simulink model "ADCS_onOrbit_14_4_3"  (R2024b)
settings: Solver=ode4  StartTime=0.0  StopTime=tspan  FixedStep=1  RelTol=1e-5
values from neighbouring files (symbols this model uses):
  A_list = [10*30; 10*30; 10*10; 10*30; 10*30; 10*10] * 1e-04    [acsLoadParameters.m]
  A_m = eye(3)    [acsLoadParameters.m]
  A_w = eye(3)    [acsLoadParameters.m]
  CD = 2.3    [acsLoadParameters.m]
  COP = [xAxis/2   0          0 ... (first row only)    [acsLoadParameters.m]
  dYear = decyear(YYYY,MM,DD)    [acsLoadParameters.m]
  e = 6.91944e-15    [acsLoadParameters.m]
  eta = 0.3    [acsLoadParameters.m]
  inc = 97.4065    [acsLoadParameters.m]
  J_body = [I_x 0 0; 0 I_y 0; 0 0 I_z]    [acsLoadParameters.m]
  J_wheels = [12894 0 0; 0 12774 0; 0 0 18389] * 1e-09    [acsLoadParameters.m]
  JD0 = juliandate(YYYY,MM,DD,HH,MIN,SEC)    [acsLoadParameters.m]
  K_d = 0.008    [acsLoadParameters.m]
  K_p = 0.003    [acsLoadParameters.m]
  K_w = 50e4    (= 500000)    [acsLoadParameters.m]
  m = 4    [acsLoadParameters.m]
  mag_moment = [0.005; 0.005; 0.005]    [acsLoadParameters.m]
  mu = 398600.4418    [acsLoadParameters.m]
  n_list = [1 0 0; 0 1 0; 0 0 1; -1 0 0; 0 -1 0; 0 0 -1]    [acsLoadParameters.m]
  omega = 0    [acsLoadParameters.m]    (also in orbit_plot_sfcn.m = block.InputPort(4).Data(:))
  p = 0.00000451    (= 4.51e-06)    [acsLoadParameters.m]    (also in cubesat_attitude_sfcn.m = ud.cubePos)
  P_0 = 0.0000001 * eye(7)    [acsLoadParameters.m]
  period = sqrt((4* pi^2 * semimajor_axis^3)/(mu))    [acsLoadParameters.m]
  q_ini = [0; 0; 0; 1]    [acsLoadParameters.m]
  raan = 132.112    [acsLoadParameters.m]
  rE = 6378.14    [acsLoadParameters.m]
  semimajor_axis = rE + h_apogee    (= 6898.14)    [acsLoadParameters.m]
  sigma_B_b = 0.05 * [1; 1; 1]    [acsLoadParameters.m]
  sigma_drift = 0.05 * [1; 1; 1] * 0    [acsLoadParameters.m]
  sigma_n = (0.05) * [1; 1; 1] * 0    [acsLoadParameters.m]
  sigma_S_b = 0.05 * [1; 1; 1]    [acsLoadParameters.m]
  tau = 300    [ATT_EKF_DOT.m]    (also in acsLoadParameters.m)
  true_anomaly = 1.42146e-14    [acsLoadParameters.m]
  w_b_ini = [0; 0.1; 0.1]    [acsLoadParameters.m]
  w_bias_0 = 0.0001 * [1; 1; 1] * 0    [acsLoadParameters.m]
  w_w_ini = [0; 0; 0]    [acsLoadParameters.m]
  wE = [0 0 15.04*(pi/180)*(1/3600)]    [acsLoadParameters.m]
undefined symbols (not defined in the file or in its folder): WMM2020
libraries: simulink_extras x13, matrix_library x9, sharedtransform x7, aerolibgravity2 x1, aerolibutil x1
(part 1 of 3)
settings Model: SimulationMode=accelerator  Creator=nimis  LastModifiedBy=nimis
settings SolverCC: AlgebraicLoopSolver=TrustRegion
settings DebuggingCC: AlgebraicLoopMsg=none

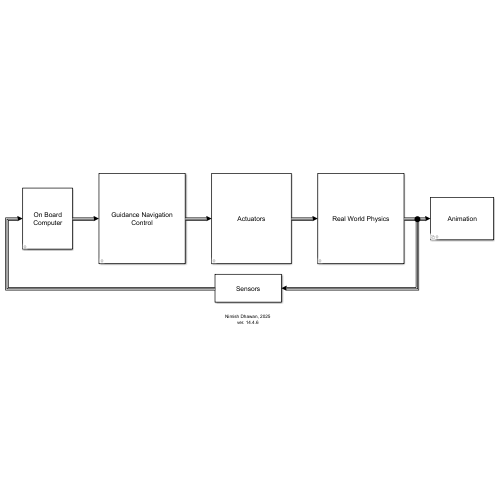
[thumbnail: Simulink's stored preview of the top-level diagram]
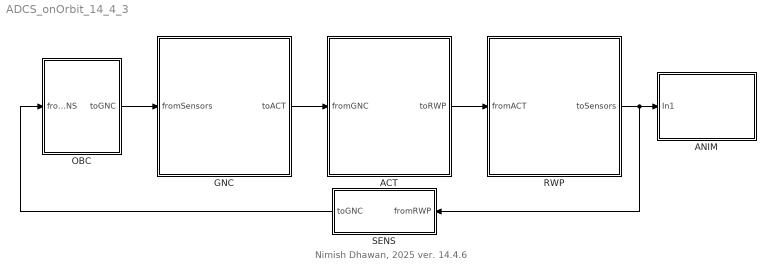
== system ADCS_onOrbit_14_4_3 ==
  note: Nimish Dhawan, 2025
      | ver. 14.4.6
  ACT : Subsystem  mask{wheel_ini=w_w_ini}
      mask prompts: wheel_ini "Wheels Initial Angular Velocity (rad/s)"
      mask DialogControl DescGroupVar Prompt: Parameters
      mask Display: disp('Actuators');
  ANIM : Subsystem  Variant=on  mask{enableAnimation=on}
      mask prompts: enableAnimation "Enable animation"
      mask DialogControl DescTextVar Prompt: Turn on or off the animation for the simulation
      mask Display: disp('Animation');
  GNC : Subsystem  mask{K_d=K_d, K_p=K_p, K_w=K_w}
      mask prompts: K_d "Controller Gain (Derivative)"; K_p "Controller Gain (Proportional)"; K_w "Controller Gain (B-dot)"
      mask DialogControl Container4 Prompt: Modified PD Controller
      mask DialogControl Container5 Prompt: B-dot Controller
      mask Display: disp('Guidance Navigation\nControl');
  OBC : Subsystem  mask{mode=Operation mode (from table)}
      mask prompts: mode "Select control mode"
      mask Display: disp('On Board\nComputer');
  RWP : Subsystem  mask{wB=w_b_ini, external_torques=on, internalProp=Internal propagator}
      mask prompts: wB "S/C Initial Angular Velocity (rad/s)"; external_torques "Enable external torques"; internalProp "Orbit Propagation"
      mask Display: disp('Real World Physics');
  SENS : Subsystem
      mask Display: disp('Sensors');
  wires:
  SENS/1(toGNC) -> OBC/1(fromSENS)
  OBC/1(toGNC) -> GNC/1(fromSensors)
  GNC/1(toACT) -> ACT/1(fromGNC)
  ACT/1(toRWP) -> RWP/1(fromACT)
  RWP/1(toSensors) -> SENS/1(fromRWP), ANIM/1(In1)

== system ADCS_onOrbit_14_4_3/ACT ==
  fromGNC : Inport
  Bus Creator : BusCreator  Inputs=3
  Bus Selector : BusSelector  OutputSignals=T_cmd,w_body,B_b,m_cmd,wheelsEnable,rodsEnable
  Demux : Demux  Outputs=3
  Demux1 : Demux  Outputs=3
  Saturation : Saturate  UpperLimit=0.2  LowerLimit=-0.2
  To Workspace : ToWorkspace  VariableName=m_1  SampleTime=-1
  To Workspace1 : ToWorkspace  VariableName=m_2  SampleTime=-1
  To Workspace10 : ToWorkspace  VariableName=h3_w  SampleTime=-1
      settings: Save2DSignal=2-D array (concatenate along first dimension)
  To Workspace11 : ToWorkspace  VariableName=h2_w  SampleTime=-1
      settings: Save2DSignal=2-D array (concatenate along first dimension)
  To Workspace12 : ToWorkspace  VariableName=h1_w  SampleTime=-1
      settings: Save2DSignal=2-D array (concatenate along first dimension)
  To Workspace2 : ToWorkspace  VariableName=m_3  SampleTime=-1
  Wheels + Magnetorquers : Subsystem
      mask Display: disp('Wheels + Magnetorquers');
  toRWP : Outport
  wires:
  Bus Selector/2 -> Wheels + Magnetorquers/2(w_b)  "<w_body>"
  Bus Selector/3 -> Wheels + Magnetorquers/3(B)  "<B_b>"
  Bus Selector/4 -> Wheels + Magnetorquers/4(m), Saturation/1  "<m_cmd>"
  Wheels + Magnetorquers/3(T_B-dot) -> Bus Creator/3  "T_B-dot"
  Demux/3 -> To Workspace10/1
  Demux/2 -> To Workspace11/1
  Wheels + Magnetorquers/2(h_w) -> Demux/1, Bus Creator/2  "h_w"
  Demux/1 -> To Workspace12/1
  Demux1/1 -> To Workspace/1
  Saturation/1 -> Demux1/1
  Demux1/2 -> To Workspace1/1
  Demux1/3 -> To Workspace2/1
  fromGNC/1 -> Bus Selector/1
  Bus Selector/1 -> Wheels + Magnetorquers/1(T_c)  "<T_cmd>"
  Bus Creator/1 -> toRWP/1
  Wheels + Magnetorquers/1(w_w) -> Bus Creator/1  "w_w"
  Bus Selector/5 -> Wheels + Magnetorquers/5(wheelsEnable)  "<wheelsEnable>"
  Bus Selector/6 -> Wheels + Magnetorquers/6(rodsEnable)  "<rodsEnable>"

== system ADCS_onOrbit_14_4_3/ANIM ==
  note: 1) Add Subsystem or Model blocks as valid variant choices.
      | 2) You cannot connect blocks at this level. At simulation, connectivity is automatically
      | determined, based on the active variant and port name matching.
  In1 : Inport
  Animation : Subsystem  VariantControl=enableAnimation == 1
  No animation : Subsystem  VariantControl=enableAnimation == 0

== system ADCS_onOrbit_14_4_3/GNC ==
  fromSensors : Inport
  Bus Creator : BusCreator  Inputs=7
  Bus Selector : BusSelector  OutputSignals=fromSENS,opMode
  Bus Selector1 : BusSelector  OutputSignals=fromSENS.state_act,fromSENS.s_I,fromSENS.r_SI,opMode
  Bus Selector2 : BusSelector  OutputSignals=fromSENS.h_w,opMode,wheelsEnable,rodsEnable
  Controller : Subsystem
      mask Display: disp('CTRL');
  Error : Subsystem
      mask Display: disp('Error');
  Guidance : Subsystem
      settings: PortSchema="{\"entries\":[{\"content\":{\"sides\":[{\"content\":{},\"type\":\"ConnectorPlacement.EquallySpacedRectSide\",\"uuid\":\"1b864df5-58d8-4c90-91c9-86121554aa4c\"},{\"content\":{\"side\":\"RIGHT\"},\"type\":\"ConnectorPlacement.EquallySpacedRectSide\",\"uuid\":\"8c8748bb-fc8a-40e3-a181-470f6593a9be\"},{\"content\":{\"connectorIds\":[\"Out1\"],\"side\":\"TOP\"},\"type\":\"ConnectorPlacement.EquallySpacedRectSide\",\"uuid\":\"61030da7-ff27-4452-a972-ecb51c641993\"},{\"content\":{\"connectorIds\":[\"In1\",\"In2\",\"In3\",\"In4\"],\"side\":\"BOTTOM\"},\"type\":\"ConnectorPlacement.EquallySpacedRectSide\",\"uuid\":\"02e92b40-894b-4184-ac6b-030597657a3a\"}]},\"type\":\"ConnectorPlacement.EquallySpacedConnector\",\"uuid\":\"ef994289-427e-4085-aff4-2d7817af2aa7\"}],\"packageUris\":[\"http://schema.mathworks.com/mf0/Connector/R2020b\"],\"version\":\"1.0\"}"
      mask Display: disp('Guidance');
  Mux : Mux  Inputs=3
  Navigation : Subsystem
      mask Display: disp('Navigation');
  Subsystem1 : Subsystem
  toACT : Outport
  wires:
  Controller/4(m) -> Bus Creator/4  "m_cmd"
  Controller/2(B_b) -> Bus Creator/2  "B_b"
  Controller/1(T_c) -> Bus Creator/1  "T_cmd"
  Bus Selector2/1 -> Controller/4(h_w)  "<h_w>"
  Controller/3(w_b) -> Bus Creator/3  "w_body"
  Error/3(delta_q) -> Subsystem1/1(In1)
  Error/2(w_error) -> Mux/2  "w_error"
  Guidance/1(desAtt) -> Error/1(desAtt)  "desAtt"
  Mux/1 -> Controller/1(error)  "error"
  Error/1(q_e) -> Mux/1  "q_errorVec"
  fromSensors/1 -> Bus Selector1/1, Bus Selector2/1, Bus Selector/1
  Bus Creator/1 -> toACT/1
  Subsystem1/1(Out1) -> Mux/3  "q_error"
  Navigation/1(w_est) -> Error/2(w_body), Controller/3(w_body)  "w_est"
  Navigation/2(q_est) -> Error/3(q_body)  "q_est"
  Navigation/3(B_est) -> Controller/2(B)  "B_est"
  Bus Selector1/1 -> Guidance/1(state)  "<state_act>"
  Bus Selector1/2 -> Guidance/2(s_I)  "<s_I>"
  Bus Selector1/3 -> Guidance/3(R_s)  "<r_SI>"
  Bus Selector1/4 -> Guidance/4(opMode)  "<opMode>"
  Bus Selector/1 -> Navigation/1(fromSENS)  "<fromSENS>"
  Bus Selector2/2 -> Bus Creator/5, Controller/5(opMode)  "<opMode>"
  Bus Selector/2 -> Navigation/2(opMode)  "<opMode>"
  Bus Selector2/3 -> Bus Creator/6  "<wheelsEnable>"
  Bus Selector2/4 -> Bus Creator/7  "<rodsEnable>"

== system ADCS_onOrbit_14_4_3/OBC ==
  fromSENS : Inport
  Bus Creator : BusCreator  Inputs=4
  Clock : Clock
  Constant : Constant  Value=mode
  From Spreadsheet : FromSpreadsheet  FileName=controlCommand.xlsx  SheetName=commands  Range=B1:E1000  InterpolationWithinTimeRange=Zero order hold  ExtrapolationAfterLastDataPoint=Hold last value
  MATLAB Function : MATLAB Function  TreatAsAtomicUnit=on
  Mux : Mux  Inputs=3
  RES : Subsystem
      mask Display: disp('Telemetry');
  toGNC : Outport
  tag scope: simTime=global
  wires:
  fromSENS/1 -> Bus Creator/1  "fromSENS"
  Bus Creator/1 -> toGNC/1
  Constant/1 -> MATLAB Function/1(internal)
  From Spreadsheet/1 -> Mux/1  "modeData"
  MATLAB Function/1(mode) -> Bus Creator/2  "opMode"
  From Spreadsheet/3 -> Mux/3  "wheelsData"
  From Spreadsheet/2 -> Mux/2  "rodsData"
  Mux/1 -> MATLAB Function/2(fromTable)
  MATLAB Function/2(wheelsEnable) -> Bus Creator/3  "wheelsEnable"
  MATLAB Function/3(rodsEnable) -> Bus Creator/4  "rodsEnable"
  Clock/1 -> [simTime]

== system ADCS_onOrbit_14_4_3/RWP ==
  fromACT : Inport
  Environment : Subsystem
      mask Display: disp('ENV');
  Nonlinear Spacecraft : Subsystem
      mask Display: image('ZLUSAT-2-3U-CubeSat-nanosatellite-model-left-system-diagram-right.png');
  Orbit Propagator : Subsystem  Variant=on
      mask Display: disp('Orbit Propagator');
  Subsystem : Subsystem
  toSensors : Outport
  wires:
  fromACT/1 -> Nonlinear Spacecraft/2(fromACT)
  Nonlinear Spacecraft/1(scOut) -> Subsystem/1(fromSC), Environment/1(scOut), Orbit Propagator/2(q_sc)
  Environment/1(envOut) -> Orbit Propagator/1(a_drag), Nonlinear Spacecraft/1(T_ext)
  Orbit Propagator/1(propOut) -> Environment/2(propIn)
  Subsystem/1(RWPoutput) -> toSensors/1

== system ADCS_onOrbit_14_4_3/SENS ==
  fromRWP : Inport
  Bus Creator : BusCreator  Inputs=10
  Bus Selector : BusSelector  OutputSignals=state,B_b,s_B,w_sc
  Bus Selector1 : BusSelector  OutputSignals=h_w,r_SI,q_sc
  Bus Selector2 : BusSelector  OutputSignals=B_I,s_I,T_ext
  GPS : Subsystem
  Gyroscope : Subsystem
  Magnetometer : Subsystem
  Sun Sensor : Subsystem
  toGNC : Outport
  wires:
  fromRWP/1 -> Bus Selector2/1, Bus Selector1/1, Bus Selector/1
  Bus Selector/1 -> GPS/1(state)  "<state>"
  GPS/1(state_act) -> Bus Creator/1  "state_act"
  Bus Selector/2 -> Magnetometer/1(B_b)  "<B_b>"
  Magnetometer/1(B_meas) -> Bus Creator/2  "B_b_meas"
  Bus Selector/3 -> Sun Sensor/1(s_B)  "<s_B>"
  Sun Sensor/1(s_B_meas) -> Bus Creator/3  "s_B_meas"
  Bus Creator/1 -> toGNC/1
  Bus Selector/4 -> Gyroscope/1(w_sc)  "<w_sc>"
  Gyroscope/1(w_meas) -> Bus Creator/4  "w_sc_meas"
  Bus Selector1/3 -> Bus Creator/7  "<q_sc>"
  Bus Selector1/2 -> Bus Creator/6  "<r_SI>"
  Bus Selector1/1 -> Bus Creator/5  "<h_w>"
  Bus Selector2/2 -> Bus Creator/9  "<s_I>"
  Bus Selector2/1 -> Bus Creator/8  "<B_I>"
  Bus Selector2/3 -> Bus Creator/10  "<T_ext>"

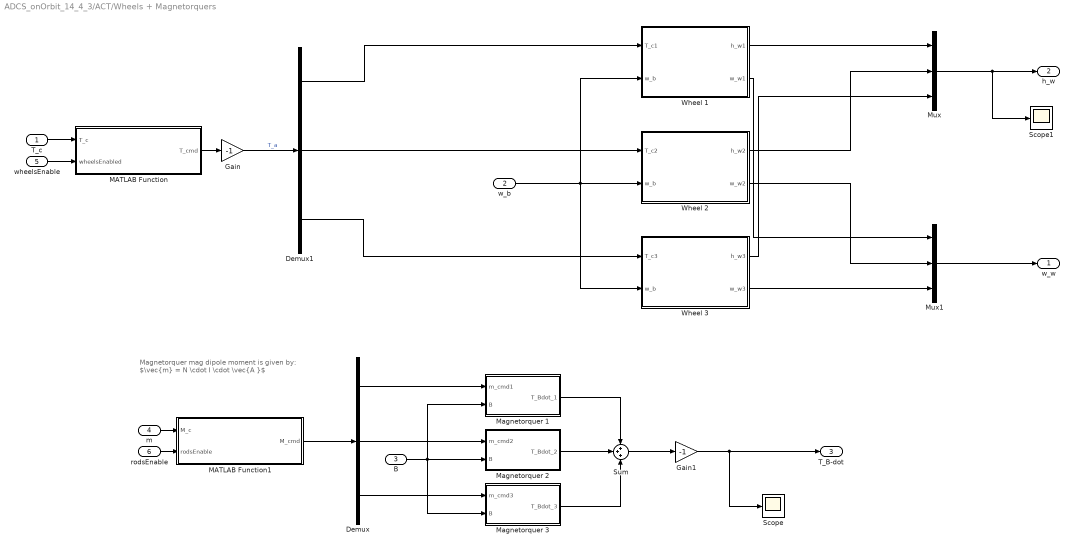
== system ADCS_onOrbit_14_4_3/ACT/Wheels + Magnetorquers ==
  note: Magnetorquer mag dipole moment is given by:
      | $\vec{m} = N \cdot I \cdot \vec{A }$
  T_c : Inport
  w_b : Inport  Port=2
  B : Inport  Port=3
  m : Inport  Port=4
  wheelsEnable : Inport  Port=5
  rodsEnable : Inport  Port=6
  Demux : Demux  Outputs=3
  Demux1 : Demux  Outputs=3
  Gain : Gain  Gain=-1
  Gain1 : Gain  Gain=-1
  MATLAB Function : MATLAB Function  TreatAsAtomicUnit=on
  MATLAB Function1 : MATLAB Function  TreatAsAtomicUnit=on
  Magnetorquer 1 : Subsystem
  Magnetorquer 2 : Subsystem
  Magnetorquer 3 : Subsystem
  Mux : Mux  Inputs=3
  Mux1 : Mux  Inputs=3
  Scope : Scope
  Scope1 : Scope
  Sum : Sum  Inputs=+++
  Wheel 1 : Subsystem
  Wheel 2 : Subsystem
  Wheel 3 : Subsystem
  w_w : Outport
  h_w : Outport  Port=2
  T_B-dot : Outport  Port=3
  wires:
  Gain/1 -> Demux1/1  "T_a"
  T_c/1 -> MATLAB Function/1(T_c)
  Demux1/1 -> Wheel 1/1(T_c1)
  Wheel 3/1(h_w3) -> Mux/3
  Wheel 1/2(w_w1) -> Mux1/1
  w_b/1 -> Wheel 3/2(w_b), Wheel 2/2(w_b), Wheel 1/2(w_b)
  Demux1/2 -> Wheel 2/1(T_c2)
  Mux/1 -> Scope1/1, h_w/1
  Wheel 1/1(h_w1) -> Mux/1
  Wheel 3/2(w_w3) -> Mux1/3
  Demux1/3 -> Wheel 3/1(T_c3)
  Wheel 2/2(w_w2) -> Mux1/2
  Gain1/1 -> T_B-dot/1, Scope/1
  Magnetorquer 3/1(T_Bdot_3) -> Sum/3
  Demux/2 -> Magnetorquer 2/1(m_cmd2)
  Magnetorquer 2/1(T_Bdot_2) -> Sum/2
  Demux/3 -> Magnetorquer 3/1(m_cmd3)
  Sum/1 -> Gain1/1
  Mux1/1 -> w_w/1
  Magnetorquer 1/1(T_Bdot_1) -> Sum/1
  B/1 -> Magnetorquer 2/2(B), Magnetorquer 3/2(B), Magnetorquer 1/2(B)
  Demux/1 -> Magnetorquer 1/1(m_cmd1)
  m/1 -> MATLAB Function1/1(M_c)
  Wheel 2/1(h_w2) -> Mux/2
  wheelsEnable/1 -> MATLAB Function/2(wheelsEnabled)
  MATLAB Function/1(T_cmd) -> Gain/1
  rodsEnable/1 -> MATLAB Function1/2(rodsEnable)
  MATLAB Function1/1(M_cmd) -> Demux/1

== system ADCS_onOrbit_14_4_3/ANIM/Animation ==
  In1 : Inport
  Bus Selector : BusSelector  OutputSignals=state
  Constant : Constant  Value=period
  Level-2 MATLAB S-Function : M-S-Function  FunctionName=orbit_plot_sfcn
  Selector : Selector  InputPortWidth=6  IndexOptions=Index vector (dialog)  Indices=[1 2 3]  OutputSizes=1
  radians2RPM : Subsystem
      mask Display:
      | port_label('output', 1, 'deg/s');
      | port_label('input', 1, 'rad/s');
  wires:
  In1/1 -> Bus Selector/1
  Selector/1 -> Level-2 MATLAB S-Function/1
  Bus Selector/1 -> Selector/1  "<state>"
  [s_I] -> Level-2 MATLAB S-Function/3
  [w_body] -> radians2RPM/1(In1)
  radians2RPM/1(Out1) -> Level-2 MATLAB S-Function/4
  Constant/1 -> Level-2 MATLAB S-Function/5
  [rpy] -> Level-2 MATLAB S-Function/2

== system ADCS_onOrbit_14_4_3/ANIM/No animation ==
  In1 : Inport
  Bus Selector : BusSelector  OutputSignals=state
  Terminator : Terminator
  wires:
  In1/1 -> Bus Selector/1
  Bus Selector/1 -> Terminator/1  "<state>"

== system ADCS_onOrbit_14_4_3/GNC/Controller ==
  error : Inport
  B : Inport  Port=2
  w_body : Inport  Port=3
  h_w : Inport  Port=4
  opMode : Inport  Port=5
  Control Algorithm : Subsystem
      mask Display: disp('Control Algorithm');
  Gain : Gain  Gain=1e-09
  Selector : Selector  InputPortWidth=10  IndexOptions=Index vector (dialog)  Indices=[1 2 3]  OutputSizes=1
  Selector1 : Selector  InputPortWidth=10  IndexOptions=Index vector (dialog)  Indices=[4 5 6]  OutputSizes=1
  Subsystem2 : Subsystem
  T_c : Outport
  B_b : Outport  Port=2
  w_b : Outport  Port=3
  m : Outport  Port=4
  wires:
  Control Algorithm/3(w_b) -> w_b/1
  Control Algorithm/2(b) -> B_b/1
  Control Algorithm/1(T_c) -> Subsystem2/1(In1)
  w_body/1 -> Control Algorithm/4(w_body)
  B/1 -> Gain/1
  Control Algorithm/4(m) -> m/1
  h_w/1 -> Control Algorithm/5(h_w)
  error/1 -> Selector1/1, Selector/1
  Selector/1 -> Control Algorithm/1(q_e)
  Selector1/1 -> Control Algorithm/2(w_error)
  Subsystem2/1(T_c) -> T_c/1
  opMode/1 -> Control Algorithm/6(opMode)
  Gain/1 -> Control Algorithm/3(B)

== system ADCS_onOrbit_14_4_3/GNC/Error ==
  desAtt : Inport
  w_body : Inport  Port=2
  q_body : Inport  Port=3
  Error Quaternion : MATLAB Function  TreatAsAtomicUnit=on
  MATLAB Function : MATLAB Function  TreatAsAtomicUnit=on
  Scope : Scope
  Selector1 : Selector  InputPortWidth=4  IndexOptions=Index vector (dialog)  Indices=[1 2 3]  OutputSizes=1
  Selector2 : Selector  InputPortWidth=7  IndexOptions=Index vector (dialog)  Indices=[1 2 3 4]  OutputSizes=1
  Selector3 : Selector  InputPortWidth=7  IndexOptions=Index vector (dialog)  Indices=[5 6 7]  OutputSizes=1
  Subsystem : Subsystem
  Sum : Sum  Inputs=|+-
  To Workspace3 : ToWorkspace  VariableName=pointing_err  SampleTime=-1
  q_e : Outport
  w_error : Outport  Port=2
  delta_q : Outport  Port=3
  wires:
  Selector2/1 -> Error Quaternion/2(q_d)
  Error Quaternion/1(delta_q) -> Subsystem/1(q), MATLAB Function/1(q_error), delta_q/1
  q_body/1 -> Error Quaternion/1(q)
  Selector1/1 -> q_e/1
  w_body/1 -> Sum/1
  Selector3/1 -> Sum/2
  Sum/1 -> w_error/1
  MATLAB Function/1(theta_e) -> To Workspace3/1, Scope/1
  desAtt/1 -> Selector3/1, Selector2/1
  Subsystem/1(Out1) -> Selector1/1

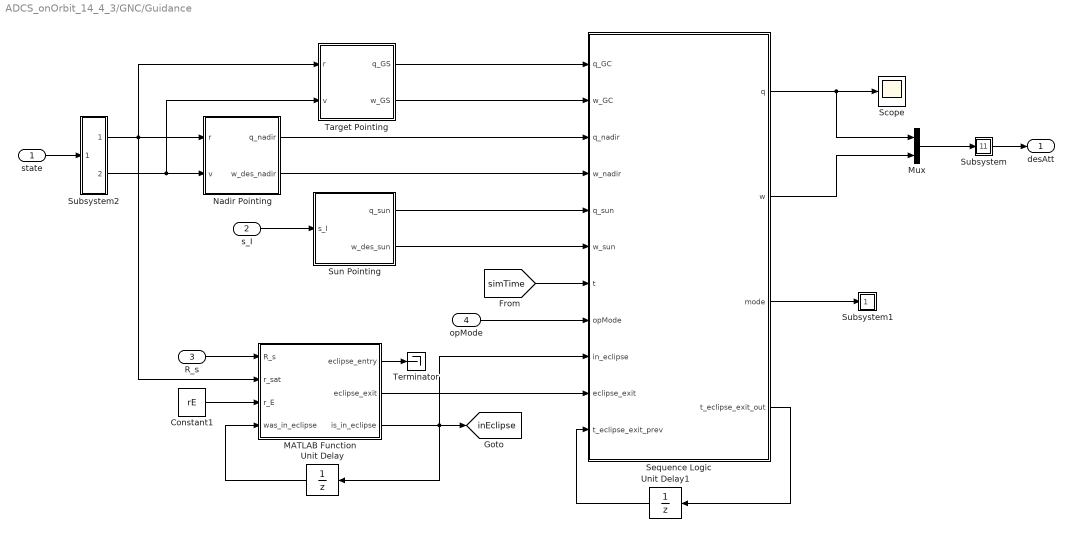
== system ADCS_onOrbit_14_4_3/GNC/Guidance ==
  state : Inport
  s_I : Inport  Port=2
  R_s : Inport  Port=3
  opMode : Inport  Port=4
  Constant1 : Constant  Value=rE
  MATLAB Function : MATLAB Function  TreatAsAtomicUnit=on
  Mux : Mux  Inputs=2
  Nadir Pointing : Subsystem
      mask Display: disp('Nadir Pointing');
  Scope : Scope
  Sequence Logic : MATLAB Function  TreatAsAtomicUnit=on
  Subsystem : Subsystem
  Subsystem1 : Subsystem
  Subsystem2 : Subsystem
      mask Display:
      | port_label('output', 1, 'r');
      | port_label('output', 2, 'v');
  Sun Pointing : Subsystem
      mask Display: disp('Sun Pointing');
  Target Pointing : Subsystem
      mask Display: disp('Target Pointing');
  Terminator : Terminator
  Unit Delay : UnitDelay  SampleTime=-1  HasFrameUpgradeWarning=on
  Unit Delay1 : UnitDelay  SampleTime=-1  HasFrameUpgradeWarning=on
  desAtt : Outport
  tag scope: inEclipse=global
  wires:
  Mux/1 -> Subsystem/1(In1)
  Sequence Logic/3(mode) -> Subsystem1/1(In1)
  Subsystem/1(Out1) -> desAtt/1
  Target Pointing/1(q_GS) -> Sequence Logic/1(q_GC)
  Target Pointing/2(w_GS) -> Sequence Logic/2(w_GC)
  R_s/1 -> MATLAB Function/1(R_s)
  opMode/1 -> Sequence Logic/8(opMode)
  MATLAB Function/3(is_in_eclipse) -> [inEclipse], Unit Delay/1, Sequence Logic/9(in_eclipse)
  Nadir Pointing/1(q_nadir) -> Sequence Logic/3(q_nadir)
  Unit Delay/1 -> MATLAB Function/4(was_in_eclipse)
  MATLAB Function/1(eclipse_entry) -> Terminator/1
  Sequence Logic/1(q) -> Mux/1, Scope/1
  [simTime] -> Sequence Logic/7(t)
  s_I/1 -> Sun Pointing/1(s_I)
  Unit Delay1/1 -> Sequence Logic/11(t_eclipse_exit_prev)
  Sun Pointing/2(w_des_sun) -> Sequence Logic/6(w_sun)
  Sequence Logic/4(t_eclipse_exit_out) -> Unit Delay1/1
  Sequence Logic/2(w) -> Mux/2
  Nadir Pointing/2(w_des_nadir) -> Sequence Logic/4(w_nadir)
  Sun Pointing/1(q_sun) -> Sequence Logic/5(q_sun)
  MATLAB Function/2(eclipse_exit) -> Sequence Logic/10(eclipse_exit)
  Constant1/1 -> MATLAB Function/3(r_E)
  Subsystem2/2(Out2) -> Target Pointing/2(v), Nadir Pointing/2(v)
  Subsystem2/1(Out1) -> MATLAB Function/2(r_sat), Target Pointing/1(r), Nadir Pointing/1(r)
  state/1 -> Subsystem2/1(In1)

== system ADCS_onOrbit_14_4_3/GNC/Navigation ==
  fromSENS : Inport
  opMode : Inport  Port=2
  Bus Selector1 : BusSelector  OutputSignals=B_b_meas
  Extended Kalman Filter : Subsystem
      mask Display: disp('EKF');
  Scope{,1..4} (5 alike) : Scope
  TRIAD Determination : Subsystem
      mask Display: disp('TRIAD');
  rad2deg : Subsystem
      mask Display:
      | port_label('output', 1, 'deg/s');
      | port_label('input', 1, 'rad/s');
  w_est : Outport
  q_est : Outport  Port=2
  B_est : Outport  Port=3
  wires:
  TRIAD Determination/1(q_det) -> Extended Kalman Filter/1(q_triad), Scope/1
  Extended Kalman Filter/2(w_est) -> w_est/1, rad2deg/1(In1)
  fromSENS/1 -> Bus Selector1/1, Extended Kalman Filter/3(fromSENS), TRIAD Determination/1(fromSENS)
  Bus Selector1/1 -> Scope3/1  "<B_b_meas>"
  opMode/1 -> Extended Kalman Filter/2(opMode)
  Extended Kalman Filter/1(q_est) -> Scope1/1, q_est/1
  Extended Kalman Filter/3(B_est) -> B_est/1, Scope4/1
  rad2deg/1(Out1) -> Scope2/1

== system ADCS_onOrbit_14_4_3/GNC/Subsystem1 ==
  In1 : Inport
  Out1 : Outport
  tag scope: q_error=global
  wires:
  In1/1 -> Out1/1, [q_error]

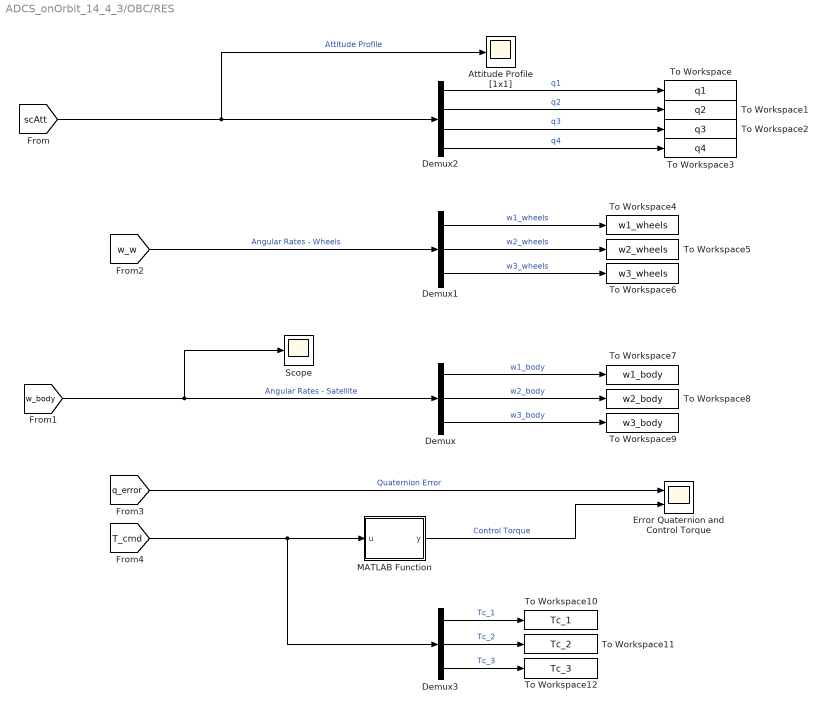
== system ADCS_onOrbit_14_4_3/OBC/RES ==
  Attitude Profile [1x1] : Scope
  Demux : Demux  Outputs=3
  Demux1 : Demux  Outputs=3
  Demux2 : Demux
  Demux3 : Demux  Outputs=3
  Error Quaternion and Control Torque : Scope  NumInputPorts=2
  MATLAB Function : MATLAB Function  TreatAsAtomicUnit=on
  Scope : Scope
  To Workspace : ToWorkspace  VariableName=q1  SampleTime=-1
      settings: Save2DSignal=2-D array (concatenate along first dimension)
  To Workspace1 : ToWorkspace  VariableName=q2  SampleTime=-1
      settings: Save2DSignal=2-D array (concatenate along first dimension)
  To Workspace10 : ToWorkspace  VariableName=Tc_1  SampleTime=-1
      settings: Save2DSignal=2-D array (concatenate along first dimension)
  To Workspace11 : ToWorkspace  VariableName=Tc_2  SampleTime=-1
      settings: Save2DSignal=2-D array (concatenate along first dimension)
  To Workspace12 : ToWorkspace  VariableName=Tc_3  SampleTime=-1
      settings: Save2DSignal=2-D array (concatenate along first dimension)
  To Workspace2 : ToWorkspace  VariableName=q3  SampleTime=-1
      settings: Save2DSignal=2-D array (concatenate along first dimension)
  To Workspace3 : ToWorkspace  VariableName=q4  SampleTime=-1
      settings: Save2DSignal=2-D array (concatenate along first dimension)
  To Workspace4 : ToWorkspace  VariableName=w1_wheels  SampleTime=-1
  To Workspace5 : ToWorkspace  VariableName=w2_wheels  SampleTime=-1
  To Workspace6 : ToWorkspace  VariableName=w3_wheels  SampleTime=-1
  To Workspace7 : ToWorkspace  VariableName=w1_body  SampleTime=-1
  To Workspace8 : ToWorkspace  VariableName=w2_body  SampleTime=-1
  To Workspace9 : ToWorkspace  VariableName=w3_body  SampleTime=-1
  wires:
  Demux1/2 -> To Workspace5/1  "w2_wheels"
  [scAtt] -> Attitude Profile [1x1]/1, Demux2/1  "Attitude Profile"
  Demux/3 -> To Workspace9/1  "w3_body"
  Demux2/3 -> To Workspace2/1  "q3"
  Demux/2 -> To Workspace8/1  "w2_body"
  MATLAB Function/1(y) -> Error Quaternion and Control Torque/2  "Control Torque"
  Demux2/2 -> To Workspace1/1  "q2"
  Demux1/3 -> To Workspace6/1  "w3_wheels"
  Demux2/1 -> To Workspace/1  "q1"
  [w_body] -> Scope/1, Demux/1  "Angular Rates - Satellite"
  Demux1/1 -> To Workspace4/1  "w1_wheels"
  Demux2/4 -> To Workspace3/1  "q4"
  Demux/1 -> To Workspace7/1  "w1_body"
  [T_cmd] -> Demux3/1, MATLAB Function/1(u)
  [w_w] -> Demux1/1  "Angular Rates - Wheels"
  Demux3/1 -> To Workspace10/1  "Tc_1"
  Demux3/2 -> To Workspace11/1  "Tc_2"
  Demux3/3 -> To Workspace12/1  "Tc_3"
  [q_error] -> Error Quaternion and Control Torque/1  "Quaternion Error"

== system ADCS_onOrbit_14_4_3/RWP/Environment ==
  scOut : Inport
  propIn : Inport  Port=2
  Bus Creator : BusCreator  Inputs=5
  Bus Selector : BusSelector  OutputSignals=s_I,state
  Bus Selector2 : BusSelector  OutputSignals=q_sc
  MATLAB Function : MATLAB Function  TreatAsAtomicUnit=on
  Quaternions to Direction Cosine Matrix : sharedtransform/Quaternions to  Direction Cosine Matrix  aMode=aMode
      settings: LibrarySourceBlock=|
      | aerolibtransform2/Quaternions to
      | Direction Cosine Matrix
  Scope : Scope
  Selector : Selector  InputPortWidth=4  IndexOptions=Index vector (dialog)  Indices=[4 1 2 3]  OutputSizes=1
  To Workspace : ToWorkspace  VariableName=T_ext  SampleTime=-1
  Variant Subsystem : Subsystem  Variant=on
  envOut : Outport
  wires:
  Variant Subsystem/3(a_drag) -> Bus Creator/3  "a_drag"
  MATLAB Function/1(y) -> Scope/1, To Workspace/1
  scOut/1 -> Bus Selector2/1
  Bus Selector/1 -> Variant Subsystem/2(s)  "<s_I>"
  Bus Selector/2 -> Variant Subsystem/3(state)  "<state>"
  Variant Subsystem/2(T_ext) -> MATLAB Function/1(u), Bus Creator/2  "T_ext"
  Variant Subsystem/1(B_b) -> Bus Creator/1  "B_b"
  Quaternions to Direction Cosine Matrix/1 -> Variant Subsystem/1(C_BI)  "C_BI"
  Selector/1 -> Quaternions to Direction Cosine Matrix/1
  Variant Subsystem/4(B_I) -> Bus Creator/4  "B_I"
  Bus Selector2/1 -> Selector/1  "<q_sc>"
  Bus Creator/1 -> envOut/1
  propIn/1 -> Bus Creator/5, Bus Selector/1  "propOut"

== system ADCS_onOrbit_14_4_3/RWP/Nonlinear Spacecraft ==
  T_ext : Inport
  fromACT : Inport  Port=2
  Bus Creator : BusCreator  Inputs=5
  Bus Selector : BusSelector  OutputSignals=T_ext
  Bus Selector1 : BusSelector  OutputSignals=h_w,T_B-dot
  Constant1 : Constant  Value=wB  VectorParams1D=off
  Scope : Scope
  Spacecraft Dynamics : Subsystem
      settings: PortSchema="{\"entries\":[{\"content\":{\"sides\":[{\"content\":{\"connectorIds\":[\"In1\",\"In2\"]},\"type\":\"ConnectorPlacement.EquallySpacedRectSide\",\"uuid\":\"7ede034c-2ba3-4dcc-9476-12360243711a\"},{\"content\":{\"connectorIds\":[\"Out1\"],\"side\":\"RIGHT\"},\"type\":\"ConnectorPlacement.EquallySpacedRectSide\",\"uuid\":\"c66fe401-c512-4312-9524-aa254a9e32f7\"},{\"content\":{\"connectorIds\":[\"In3\",\"In4\"],\"side\":\"TOP\"},\"type\":\"ConnectorPlacement.EquallySpacedRectSide\",\"uuid\":\"402e5e38-17e5-4915-9174-3100d56d3172\"}]},\"type\":\"ConnectorPlacement.EquallySpacedConnector\",\"uuid\":\"b1776140-59a6-461e-842e-8039fbfbf661\"}],\"packageUris\":[\"http://schema.mathworks.com/mf0/Connector/R2020b\"],\"version\":\"1.0\"}"
  Spacecraft Kinematics : Subsystem
      settings: PortSchema="{\"entries\":[{\"content\":{\"sides\":[{\"content\":{\"connectorIds\":[\"In1\"]},\"type\":\"ConnectorPlacement.EquallySpacedRectSide\",\"uuid\":\"794d76cd-b5e7-4ff8-8068-00704bd683ee\"},{\"content\":{\"connectorIds\":[\"Out1\"],\"side\":\"RIGHT\"},\"type\":\"ConnectorPlacement.EquallySpacedRectSide\",\"uuid\":\"8689c2da-569a-445b-beb1-f77a8b01ef76\"},{\"content\":{\"connectorIds\":[\"In2\"],\"side\":\"TOP\"},\"type\":\"ConnectorPlacement.EquallySpacedRectSide\",\"uuid\":\"54cd84e3-9f07-4737-bd46-1b0993503ebe\"}]},\"type\":\"ConnectorPlacement.EquallySpacedConnector\",\"uuid\":\"d9405558-e6b2-41dd-b599-a734e1169741\"}],\"packageUris\":[\"http://schema.mathworks.com/mf0/Connector/R2020b\"],\"version\":\"1.0\"}"
  Subsystem : Subsystem
  q_sat_ini : Constant  Value=q_ini  VectorParams1D=off
  scOut : Outport
  wires:
  q_sat_ini/1 -> Spacecraft Kinematics/2(q_ini)
  T_ext/1 -> Bus Creator/4, Bus Selector/1  "envOut"
  Bus Selector1/2 -> Spacecraft Dynamics/2(T_Bdot)  "<T_B-dot>"
  fromACT/1 -> Bus Creator/5, Bus Selector1/1  "fromACT"
  Constant1/1 -> Spacecraft Dynamics/4(w_sat_ini)
  Spacecraft Kinematics/1(q) -> Scope/1, Subsystem/1(q)
  Spacecraft Dynamics/1(w_b) -> Bus Creator/2, Spacecraft Kinematics/1(w)  "w_sc"
  Bus Creator/1 -> scOut/1
  Bus Selector/1 -> Spacecraft Dynamics/3(T_b)  "<T_ext>"
  Bus Selector1/1 -> Bus Creator/3, Spacecraft Dynamics/1(h_w)  "<h_w>"
  Subsystem/1(Out1) -> Bus Creator/1  "q_sc"

== system ADCS_onOrbit_14_4_3/RWP/Orbit Propagator ==
  note: 1) Add Subsystem or Model blocks as valid variant choices.
      | 2) You cannot connect blocks at this level. At simulation, connectivity is automatically
      | determined, based on the active variant and port name matching.
  a_drag : Inport
  q_sc : Inport  Port=2
  External : Subsystem  VariantControl=internalProp == 0
  Internal : Subsystem  VariantControl=internalProp == 1
  propOut : Outport

== system ADCS_onOrbit_14_4_3/RWP/Subsystem ==
  fromSC : Inport
  Bus Creator : BusCreator  Inputs=11
  Bus Selector2 : BusSelector  OutputSignals=q_sc,w_sc,envOut,fromACT.h_w,fromACT.w_w
  Bus Selector3 : BusSelector  OutputSignals=B_I,B_b,T_ext,propOut
  Bus Selector4 : BusSelector  OutputSignals=s_I,state,s_B,r_SI
  Subsystem1 : Subsystem
  Subsystem2 : Subsystem
  RWPoutput : Outport
  wires:
  Subsystem1/1(Out1) -> Bus Creator/11  "w_w"
  Bus Selector4/3 -> Bus Creator/8  "<s_B>"
  Bus Selector3/4 -> Bus Selector4/1  "<propOut>"
  Bus Selector3/2 -> Bus Creator/4  "<B_b>"
  Subsystem2/1(Out1) -> Bus Creator/6  "s_I"
  Bus Selector2/3 -> Bus Selector3/1  "<envOut>"
  Bus Selector4/2 -> Bus Creator/7  "<state>"
  Bus Selector4/4 -> Bus Creator/9  "<r_SI>"
  Bus Selector2/2 -> Bus Creator/2  "<w_sc>"
  Bus Selector4/1 -> Subsystem2/1(In1)  "<s_I>"
  Bus Selector3/1 -> Bus Creator/3  "<B_I>"
  Bus Selector2/1 -> Bus Creator/1  "<q_sc>"
  Bus Creator/1 -> RWPoutput/1
  fromSC/1 -> Bus Selector2/1
  Bus Selector3/3 -> Bus Creator/5  "<T_ext>"
  Bus Selector2/4 -> Bus Creator/10  "<h_w>"
  Bus Selector2/5 -> Subsystem1/1(In1)  "<w_w>"

== system ADCS_onOrbit_14_4_3/SENS/GPS ==
  state : Inport
  state_act : Outport
  wires:
  state/1 -> state_act/1

== system ADCS_onOrbit_14_4_3/SENS/Gyroscope ==
  note: Switch down sends angular velocity values with
      | noise and bias. Make sure to nullify the variances
      | when not using the gyro estimation.
  w_sc : Inport
  Integrator : Integrator  InitialCondition=w_bias_0
  MATLAB Function : MATLAB Function  TreatAsAtomicUnit=on
  MATLAB Function1 : MATLAB Function  TreatAsAtomicUnit=on
  Manual Switch : ManualSwitch
  Random Number3 : RandomNumber  Variance=2*((0.05*pi/180)^2)/300  Seed=123  SampleTime=1
  Random Number4 : RandomNumber  Variance=(0.05*pi/180)^2  SampleTime=1
  w_meas : Outport
  wires:
  w_sc/1 -> Manual Switch/1, MATLAB Function1/1(w_sc)
  MATLAB Function/1(biasDot) -> Integrator/1
  Random Number3/1 -> MATLAB Function/2(noise)
  Integrator/1 -> MATLAB Function1/2(bias), MATLAB Function/1(bias)
  Random Number4/1 -> MATLAB Function1/3(noise)
  MATLAB Function1/1(w_meas) -> Manual Switch/2
  Manual Switch/1 -> w_meas/1

== system ADCS_onOrbit_14_4_3/SENS/Magnetometer ==
  B_b : Inport
  Demux : Demux  Outputs=3
  Manual Switch : ManualSwitch
  Mux : Mux  Inputs=3
  Random Number : RandomNumber  Variance=0.05^2  Seed=123  SampleTime=1
  Random Number1 : RandomNumber  Variance=0.05^2  Seed=123  SampleTime=1
  Random Number2 : RandomNumber  Variance=0.05^2  Seed=123  SampleTime=1
  Sum : Sum  Inputs=|++
  Sum1 : Sum  Inputs=|++
  Sum2 : Sum  Inputs=|++
  B_meas : Outport
  wires:
  Mux/1 -> Manual Switch/1
  Sum2/1 -> Mux/3
  Random Number/1 -> Sum/2
  Random Number1/1 -> Sum1/2
  Demux/3 -> Sum2/1
  Demux/2 -> Sum1/1
  Sum1/1 -> Mux/2
  Demux/1 -> Sum/1
  B_b/1 -> Manual Switch/2, Demux/1
  Sum/1 -> Mux/1
  Random Number2/1 -> Sum2/2
  Manual Switch/1 -> B_meas/1

== system ADCS_onOrbit_14_4_3/SENS/Sun Sensor ==
  note: This assumes that the sun sensor reference frame coincides
      | with the sc body reference frame
  s_B : Inport
  Demux : Demux  Outputs=3
  Manual Switch : ManualSwitch
  Mux : Mux  Inputs=3
  Random Number : RandomNumber  Variance=0.001^2  SampleTime=1
  Random Number1 : RandomNumber  Variance=0.001^2  SampleTime=1
  Random Number2 : RandomNumber  Variance=0.001^2  SampleTime=1
  Sum : Sum  Inputs=|++
  Sum1 : Sum  Inputs=|++
  Sum2 : Sum  Inputs=|++
  s_B_meas : Outport
  wires:
  Demux/1 -> Sum/1
  Random Number/1 -> Sum/2
  Demux/2 -> Sum1/1
  Random Number1/1 -> Sum1/2
  Demux/3 -> Sum2/1
  Random Number2/1 -> Sum2/2
  Sum/1 -> Mux/1
  Sum1/1 -> Mux/2
  Sum2/1 -> Mux/3
  s_B/1 -> Manual Switch/2, Demux/1
  Mux/1 -> Manual Switch/1
  Manual Switch/1 -> s_B_meas/1

== system ADCS_onOrbit_14_4_3/ACT/Wheels + Magnetorquers/Magnetorquer 1 ==
  m_cmd1 : Inport
  B : Inport  Port=2
  Constant1 : Constant  Value=A_m
  Matrix Multiply : Product
  Matrix Multiply1 : Product  Multiplication=Matrix(*)
  Saturation : Saturate  UpperLimit=0.2  LowerLimit=-0.2
  Submatrix : matrix_library/Submatrix  RowSpan=One row  RowStartMode=Index  RowStartIndex=1  RowEndMode=Last  RowEndIndex=1  ColSpan=All columns  ColStartMode=First  ColStartIndex=1  ColEndMode=Last  ColEndIndex=1
  Transpose : Math  Operator=transpose
  skew symmetric : MATLAB Function  TreatAsAtomicUnit=on
  T_Bdot_1 : Outport
  wires:
  Constant1/1 -> Submatrix/1
  skew symmetric/1(skew) -> Matrix Multiply1/1
  Matrix Multiply1/1 -> T_Bdot_1/1
  Submatrix/1 -> Transpose/1
  Matrix Multiply/1 -> skew symmetric/1(M)
  B/1 -> Matrix Multiply1/2
  Transpose/1 -> Matrix Multiply/2
  m_cmd1/1 -> Saturation/1
  Saturation/1 -> Matrix Multiply/1

== system ADCS_onOrbit_14_4_3/ACT/Wheels + Magnetorquers/Magnetorquer 2 ==
  m_cmd2 : Inport
  B : Inport  Port=2
  Constant1 : Constant  Value=A_m
  Display : Display
  Display1 : Display
  Matrix Multiply : Product
  Matrix Multiply1 : Product  Multiplication=Matrix(*)
  Saturation : Saturate  UpperLimit=0.2  LowerLimit=-0.2
  Submatrix : matrix_library/Submatrix  RowSpan=One row  RowStartMode=Index  RowStartIndex=2  RowEndMode=Last  RowEndIndex=1  ColSpan=All columns  ColStartMode=First  ColStartIndex=1  ColEndMode=Last  ColEndIndex=1
  Transpose : Math  Operator=transpose
  skew symmetric : MATLAB Function  TreatAsAtomicUnit=on
  T_Bdot_2 : Outport
  wires:
  m_cmd2/1 -> Saturation/1
  Transpose/1 -> Matrix Multiply/2
  B/1 -> Matrix Multiply1/2
  Matrix Multiply/1 -> skew symmetric/1(M), Display/1
  Submatrix/1 -> Transpose/1
  Matrix Multiply1/1 -> Display1/1, T_Bdot_2/1
  skew symmetric/1(skew) -> Matrix Multiply1/1
  Constant1/1 -> Submatrix/1
  Saturation/1 -> Matrix Multiply/1

== system ADCS_onOrbit_14_4_3/ACT/Wheels + Magnetorquers/Magnetorquer 3 ==
  m_cmd3 : Inport
  B : Inport  Port=2
  Constant1 : Constant  Value=A_m
  Display : Display
  Display1 : Display
  Matrix Multiply : Product
  Matrix Multiply1 : Product  Multiplication=Matrix(*)
  Saturation : Saturate  UpperLimit=0.2  LowerLimit=-0.2
  Submatrix : matrix_library/Submatrix  RowSpan=One row  RowStartMode=Index  RowStartIndex=3  RowEndMode=Last  RowEndIndex=1  ColSpan=All columns  ColStartMode=First  ColStartIndex=1  ColEndMode=Last  ColEndIndex=1
  Transpose : Math  Operator=transpose
  skew symmetric : MATLAB Function  TreatAsAtomicUnit=on
  T_Bdot_3 : Outport
  wires:
  Constant1/1 -> Submatrix/1
  skew symmetric/1(skew) -> Matrix Multiply1/1
  Matrix Multiply1/1 -> T_Bdot_3/1, Display1/1
  Submatrix/1 -> Transpose/1
  Matrix Multiply/1 -> skew symmetric/1(M), Display/1
  B/1 -> Matrix Multiply1/2
  Transpose/1 -> Matrix Multiply/2
  m_cmd3/1 -> Saturation/1
  Saturation/1 -> Matrix Multiply/1

== system ADCS_onOrbit_14_4_3/ACT/Wheels + Magnetorquers/Wheel 1 ==
  note: $\vec{\omega_{w}} = \textbf{J}_w^{-1}\vec{h_w} - \textbf{A}_w \vec{\omega_b}$
  T_c1 : Inport
  w_b : Inport  Port=2
  " w_w" : Constant  Value=wheel_ini  VectorParams1D=off
  Constant : Constant  Value=J_wheels  VectorParams1D=off
  Constant1 : Constant  Value=A_w
  Integrator : Integrator  InitialConditionSource=external
  MATLAB Function : MATLAB Function  TreatAsAtomicUnit=on
  Matrix Multiply : Product
  Matrix Multiply1 : Product  Multiplication=Matrix(*)
  Matrix Multiply2 : Product
  Selector1 : Selector  InputPortWidth=3  IndexOptions=Index vector (dialog)  Indices=[1]  OutputSizes=1
  Submatrix : matrix_library/Submatrix  RowSpan=One row  RowStartMode=Index  RowStartIndex=1  RowEndMode=Last  RowEndIndex=1  ColSpan=All columns  ColStartMode=First  ColStartIndex=1  ColEndMode=Last  ColEndIndex=1
  Submatrix1 : matrix_library/Submatrix  RowSpan=One row  RowStartMode=Index  RowStartIndex=3  RowEndMode=Last  RowEndIndex=1  ColSpan=One column  ColStartMode=Index  ColStartIndex=3  ColEndMode=Last  ColEndIndex=1
  Sum : Sum  Inputs=|+-
  h_w1 : Outport
  w_w1 : Outport  Port=2
  wires:
  Integrator/1 -> Matrix Multiply/2, h_w1/1  "h_w"
  w_b/1 -> Matrix Multiply1/2
  Sum/1 -> w_w1/1  "w_w"
  Matrix Multiply1/1 -> Sum/2  "J_w_inv.h_w"
  Matrix Multiply2/1 -> Integrator/2
  Constant1/1 -> Submatrix/1
  Matrix Multiply/1 -> Sum/1  "J_w_inv.h_w"
  Constant/1 -> Submatrix1/1
  T_c1/1 -> Integrator/1
  " w_w"/1 -> Selector1/1
  Submatrix/1 -> Matrix Multiply1/1
  Submatrix1/1 -> Matrix Multiply2/1, MATLAB Function/1(u)
  MATLAB Function/1(y) -> Matrix Multiply/1
  Selector1/1 -> Matrix Multiply2/2

== system ADCS_onOrbit_14_4_3/ACT/Wheels + Magnetorquers/Wheel 2 ==
  note: $\vec{\omega_{w}} = \textbf{J}_w^{-1}\vec{h_w} - \textbf{A}_w \vec{\omega_b}$
  T_c2 : Inport
  w_b : Inport  Port=2
  " w_w" : Constant  Value=wheel_ini  VectorParams1D=off
  Constant : Constant  Value=J_wheels  VectorParams1D=off
  Constant1 : Constant  Value=A_w
  Integrator : Integrator  InitialConditionSource=external
  MATLAB Function : MATLAB Function  TreatAsAtomicUnit=on
  Matrix Multiply : Product
  Matrix Multiply1 : Product  Multiplication=Matrix(*)
  Matrix Multiply2 : Product
  Selector1 : Selector  InputPortWidth=3  IndexOptions=Index vector (dialog)  Indices=[2]  OutputSizes=1
  Submatrix1 : matrix_library/Submatrix  RowSpan=One row  RowStartMode=Index  RowStartIndex=3  RowEndMode=Last  RowEndIndex=1  ColSpan=One column  ColStartMode=Index  ColStartIndex=3  ColEndMode=Last  ColEndIndex=1
  Submatrix2 : matrix_library/Submatrix  RowSpan=One row  RowStartMode=Index  RowStartIndex=2  RowEndMode=Last  RowEndIndex=1  ColSpan=All columns  ColStartMode=First  ColStartIndex=1  ColEndMode=Last  ColEndIndex=1
  Sum : Sum  Inputs=|+-
  h_w2 : Outport
  w_w2 : Outport  Port=2
  wires:
  Selector1/1 -> Matrix Multiply2/2
  MATLAB Function/1(y) -> Matrix Multiply/1
  Submatrix1/1 -> MATLAB Function/1(u), Matrix Multiply2/1
  Submatrix2/1 -> Matrix Multiply1/1
  " w_w"/1 -> Selector1/1
  T_c2/1 -> Integrator/1
  Constant/1 -> Submatrix1/1
  Matrix Multiply/1 -> Sum/1  "J_w_inv.h_w"
  Constant1/1 -> Submatrix2/1
  Matrix Multiply2/1 -> Integrator/2
  Matrix Multiply1/1 -> Sum/2  "J_w_inv.h_w"
  Sum/1 -> w_w2/1  "w_w"
  w_b/1 -> Matrix Multiply1/2
  Integrator/1 -> h_w2/1, Matrix Multiply/2  "h_w"

== system ADCS_onOrbit_14_4_3/ACT/Wheels + Magnetorquers/Wheel 3 ==
  note: $\vec{\omega_{w}} = \textbf{J}_w^{-1}\vec{h_w} - \textbf{A}_w \vec{\omega_b}$
  T_c3 : Inport
  w_b : Inport  Port=2
  " w_w" : Constant  Value=wheel_ini  VectorParams1D=off
  Constant : Constant  Value=J_wheels  VectorParams1D=off
  Constant1 : Constant  Value=A_w
  Integrator : Integrator  InitialConditionSource=external
  MATLAB Function : MATLAB Function  TreatAsAtomicUnit=on
  Matrix Multiply : Product
  Matrix Multiply1 : Product  Multiplication=Matrix(*)
  Matrix Multiply2 : Product
  Selector1 : Selector  InputPortWidth=3  IndexOptions=Index vector (dialog)  Indices=[3]  OutputSizes=1
  Submatrix1 : matrix_library/Submatrix  RowSpan=One row  RowStartMode=Index  RowStartIndex=3  RowEndMode=Last  RowEndIndex=1  ColSpan=One column  ColStartMode=Index  ColStartIndex=3  ColEndMode=Last  ColEndIndex=1
  Submatrix2 : matrix_library/Submatrix  RowSpan=One row  RowStartMode=Index  RowStartIndex=3  RowEndMode=Last  RowEndIndex=1  ColSpan=All columns  ColStartMode=First  ColStartIndex=1  ColEndMode=Last  ColEndIndex=1
  Sum : Sum  Inputs=|+-
  h_w3 : Outport
  w_w3 : Outport  Port=2
  wires:
  Integrator/1 -> Matrix Multiply/2, h_w3/1  "h_w"
  w_b/1 -> Matrix Multiply1/2
  Sum/1 -> w_w3/1  "w_w"
  Matrix Multiply1/1 -> Sum/2  "J_w_inv.h_w"
  Matrix Multiply2/1 -> Integrator/2
  Constant1/1 -> Submatrix2/1
  Matrix Multiply/1 -> Sum/1  "J_w_inv.h_w"
  Constant/1 -> Submatrix1/1
  T_c3/1 -> Integrator/1
  " w_w"/1 -> Selector1/1
  Submatrix2/1 -> Matrix Multiply1/1
  Submatrix1/1 -> Matrix Multiply2/1, MATLAB Function/1(u)
  MATLAB Function/1(y) -> Matrix Multiply/1
  Selector1/1 -> Matrix Multiply2/2

== system ADCS_onOrbit_14_4_3/ANIM/Animation/radians2RPM ==
  In1 : Inport
  Gain : Gain  Gain=57.2958
  Out1 : Outport
  wires:
  In1/1 -> Gain/1
  Gain/1 -> Out1/1

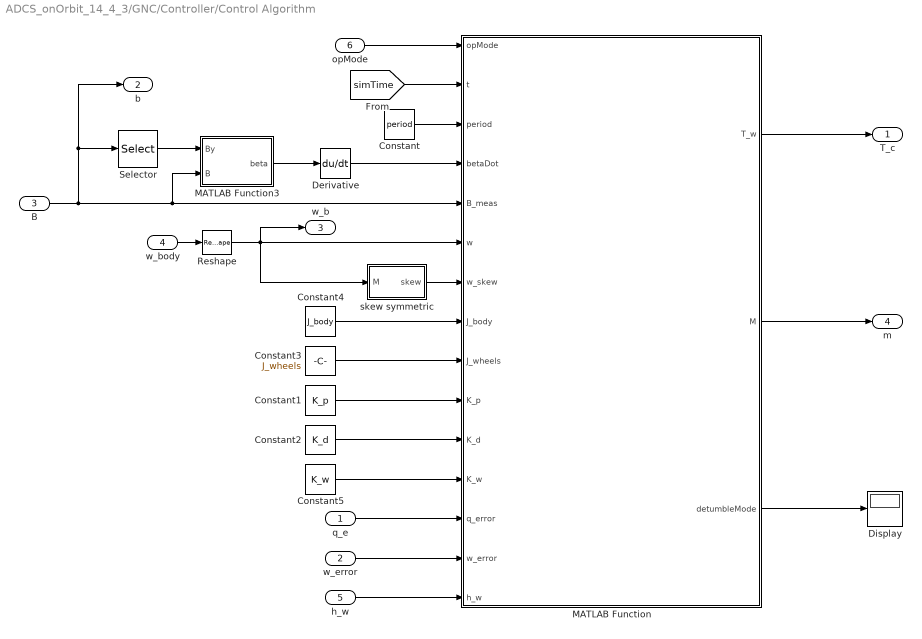
== system ADCS_onOrbit_14_4_3/GNC/Controller/Control Algorithm ==
  q_e : Inport
  w_error : Inport  Port=2
  B : Inport  Port=3
  w_body : Inport  Port=4
  h_w : Inport  Port=5
  opMode : Inport  Port=6
  Constant : Constant  Value=period
  Constant1 : Constant  Value=K_p
  Constant2 : Constant  Value=K_d
  Constant3 : Constant  Value=J_wheels
  Constant4 : Constant  Value=J_body
  Constant5 : Constant  Value=K_w
  Derivative : Derivative
  Display : Display
  MATLAB Function : MATLAB Function  TreatAsAtomicUnit=on
  MATLAB Function3 : MATLAB Function  TreatAsAtomicUnit=on
  Reshape : Reshape  OutputDimensionality=Customize  OutputDimensions=[3,1]
  Selector : Selector  InputPortWidth=3  IndexOptions=Index vector (dialog)  Indices=[2]  OutputSizes=1
  skew symmetric : MATLAB Function  TreatAsAtomicUnit=on
  T_c : Outport
  b : Outport  Port=2
  w_b : Outport  Port=3
  m : Outport  Port=4
  wires:
  Constant/1 -> MATLAB Function/3(period)
  MATLAB Function/3(detumbleMode) -> Display/1
  MATLAB Function/2(M) -> m/1
  Derivative/1 -> MATLAB Function/4(betaDot)
  h_w/1 -> MATLAB Function/15(h_w)
  Constant3/1 -> MATLAB Function/9(J_wheels)
  w_body/1 -> Reshape/1
  B/1 -> b/1, Selector/1, MATLAB Function3/2(B), MATLAB Function/5(B_meas)
  w_error/1 -> MATLAB Function/14(w_error)
  q_e/1 -> MATLAB Function/13(q_error)
  [simTime] -> MATLAB Function/2(t)
  Selector/1 -> MATLAB Function3/1(By)
  Constant4/1 -> MATLAB Function/8(J_body)
  MATLAB Function3/1(beta) -> Derivative/1
  Constant1/1 -> MATLAB Function/10(K_p)
  MATLAB Function/1(T_w) -> T_c/1
  Constant2/1 -> MATLAB Function/11(K_d)
  skew symmetric/1(skew) -> MATLAB Function/7(w_skew)
  Constant5/1 -> MATLAB Function/12(K_w)
  opMode/1 -> MATLAB Function/1(opMode)
  Reshape/1 -> MATLAB Function/6(w), skew symmetric/1(M), w_b/1

== system ADCS_onOrbit_14_4_3/GNC/Controller/Subsystem2 ==
  In1 : Inport
  T_c : Outport
  tag scope: T_cmd=global
  wires:
  In1/1 -> T_c/1, [T_cmd]

== system ADCS_onOrbit_14_4_3/GNC/Error/Subsystem ==
  q : Inport
  MATLAB Function1 : MATLAB Function  TreatAsAtomicUnit=on
  Radians to Degrees : simulink_extras/Transformations/Radians to Degrees
  Radians to Degrees1 : simulink_extras/Transformations/Radians to Degrees
  Radians to Degrees2 : simulink_extras/Transformations/Radians to Degrees
  To Workspace : ToWorkspace  VariableName=roll_err  SampleTime=-1
  To Workspace1 : ToWorkspace  VariableName=pitch_err  SampleTime=-1
  To Workspace2 : ToWorkspace  VariableName=yaw_err  SampleTime=-1
  Out1 : Outport
  wires:
  q/1 -> MATLAB Function1/1(q), Out1/1
  MATLAB Function1/2(pitch) -> Radians to Degrees1/1
  Radians to Degrees2/1 -> To Workspace2/1
  Radians to Degrees/1 -> To Workspace/1
  MATLAB Function1/3(yaw) -> Radians to Degrees2/1
  MATLAB Function1/1(roll) -> Radians to Degrees/1
  Radians to Degrees1/1 -> To Workspace1/1

== system ADCS_onOrbit_14_4_3/GNC/Guidance/Nadir Pointing ==
  r : Inport
  v : Inport  Port=2
  Constant : Constant  Value=[0; -0.001108; 0]  VectorParams1D=off
  Direction Cosine Matrix to Quaternions : sharedtransform/Direction Cosine Matrix  to Quaternions  aMode=0  action=None  tolerance=eps(2)
      settings: LibrarySourceBlock=|
      | aerolibtransform2/Direction Cosine Matrix
      | to Quaternions
  ECI to SB : MATLAB Function  TreatAsAtomicUnit=on
  Quaternion Continuity : Subsystem
      mask Display: disp('Quaternion\nContinuity');
  Selector2 : Selector  InputPortWidth=4  IndexOptions=Index vector (dialog)  Indices=[2 3 4 1]  OutputSizes=1
  q_nadir : Outport
  w_des_nadir : Outport  Port=2
  wires:
  v/1 -> ECI to SB/2(v)
  r/1 -> ECI to SB/1(r)
  Constant/1 -> w_des_nadir/1
  Direction Cosine Matrix to Quaternions/1 -> Selector2/1
  ECI to SB/1(C_BI) -> Direction Cosine Matrix to Quaternions/1
  Selector2/1 -> Quaternion Continuity/1(q)
  Quaternion Continuity/1(q_smooth) -> q_nadir/1

== system ADCS_onOrbit_14_4_3/GNC/Guidance/Subsystem ==
  In1 : Inport
  Demux2 : Demux
  Selector : Selector  InputPortWidth=7  IndexOptions=Index vector (dialog)  Indices=[1 2 3 4]  OutputSizes=1
  To Workspace : ToWorkspace  VariableName=q1_des  SampleTime=-1
      settings: Save2DSignal=2-D array (concatenate along first dimension)
  To Workspace1 : ToWorkspace  VariableName=q2_des  SampleTime=-1
      settings: Save2DSignal=2-D array (concatenate along first dimension)
  To Workspace2 : ToWorkspace  VariableName=q3_des  SampleTime=-1
      settings: Save2DSignal=2-D array (concatenate along first dimension)
  To Workspace3 : ToWorkspace  VariableName=q4_des  SampleTime=-1
      settings: Save2DSignal=2-D array (concatenate along first dimension)
  Out1 : Outport
  wires:
  Selector/1 -> Demux2/1
  Demux2/1 -> To Workspace/1  "q1_des"
  Demux2/2 -> To Workspace1/1  "q2_des"
  Demux2/3 -> To Workspace2/1  "q3_des"
  In1/1 -> Selector/1, Out1/1
  Demux2/4 -> To Workspace3/1  "q4_des"

== system ADCS_onOrbit_14_4_3/GNC/Guidance/Subsystem1 ==
  In1 : Inport
  To Workspace4 : ToWorkspace  VariableName=mode  SampleTime=-1
      settings: Save2DSignal=2-D array (concatenate along first dimension)
  wires:
  In1/1 -> To Workspace4/1

== system ADCS_onOrbit_14_4_3/GNC/Guidance/Subsystem2 ==
  In1 : Inport
  Selector1 : Selector  InputPortWidth=6  IndexOptions=Index vector (dialog)  Indices=[1 2 3]  OutputSizes=1
  Selector2 : Selector  InputPortWidth=6  IndexOptions=Index vector (dialog)  Indices=[4 5 6]  OutputSizes=1
  Out1 : Outport
  Out2 : Outport  Port=2
  wires:
  Selector1/1 -> Out1/1
  In1/1 -> Selector2/1, Selector1/1
  Selector2/1 -> Out2/1

== system ADCS_onOrbit_14_4_3/GNC/Guidance/Sun Pointing ==
  s_I : Inport
  Constant : Constant  Value=[0;0;0]  VectorParams1D=off
  MATLAB Function : MATLAB Function  TreatAsAtomicUnit=on
  MATLAB Function2 : MATLAB Function  TreatAsAtomicUnit=on
  Quaternion Continuity : Subsystem
      mask Display: disp('Quaternion\nContinuity');
  q_sun : Outport
  w_des_sun : Outport  Port=2
  wires:
  s_I/1 -> MATLAB Function2/1(s_i)
  MATLAB Function2/1(C_BI) -> MATLAB Function/1(DCM)
  Constant/1 -> w_des_sun/1
  MATLAB Function/1(q) -> Quaternion Continuity/1(q)
  Quaternion Continuity/1(q_smooth) -> q_sun/1

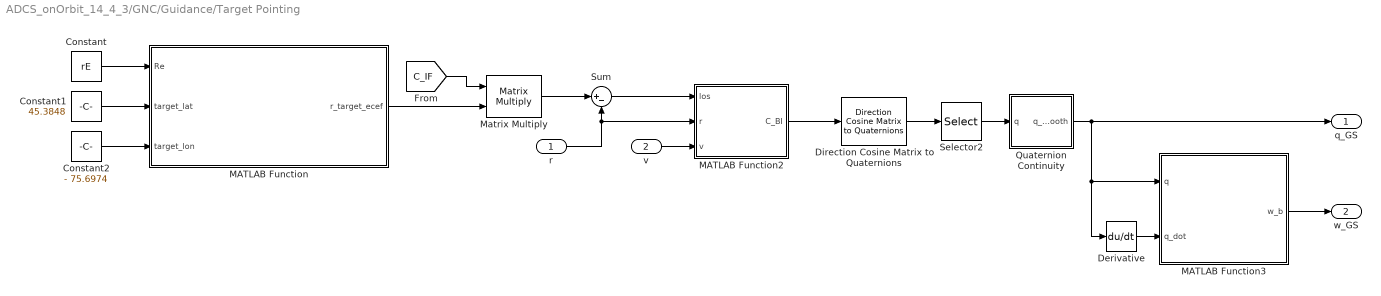
== system ADCS_onOrbit_14_4_3/GNC/Guidance/Target Pointing ==
  r : Inport
  v : Inport  Port=2
  Constant : Constant  Value=rE
  Constant1 : Constant  Value=45.3848
  Constant2 : Constant  Value=- 75.6974
  Derivative : Derivative
  Direction Cosine Matrix to Quaternions : sharedtransform/Direction Cosine Matrix  to Quaternions  aMode=0  action=None  tolerance=eps(2)
      settings: LibrarySourceBlock=|
      | aerolibtransform2/Direction Cosine Matrix
      | to Quaternions
  MATLAB Function : MATLAB Function  TreatAsAtomicUnit=on
  MATLAB Function2 : MATLAB Function  TreatAsAtomicUnit=on
  MATLAB Function3 : MATLAB Function  TreatAsAtomicUnit=on
  Matrix Multiply : Product  Multiplication=Matrix(*)
  Quaternion Continuity : Subsystem
      mask Display: disp('Quaternion\nContinuity');
  Selector2 : Selector  InputPortWidth=4  IndexOptions=Index vector (dialog)  Indices=[2 3 4 1]  OutputSizes=1
  Sum : Sum  Inputs=|+-
  q_GS : Outport
  w_GS : Outport  Port=2
  wires:
  Constant/1 -> MATLAB Function/1(Re)
  Constant1/1 -> MATLAB Function/2(target_lat)
  Constant2/1 -> MATLAB Function/3(target_lon)
  MATLAB Function/1(r_target_ecef) -> Matrix Multiply/2
  Matrix Multiply/1 -> Sum/1
  r/1 -> MATLAB Function2/2(r), Sum/2
  Sum/1 -> MATLAB Function2/1(los)
  MATLAB Function2/1(C_BI) -> Direction Cosine Matrix to Quaternions/1
  Direction Cosine Matrix to Quaternions/1 -> Selector2/1
  Selector2/1 -> Quaternion Continuity/1(q)
  Quaternion Continuity/1(q_smooth) -> Derivative/1, MATLAB Function3/1(q), q_GS/1
  Derivative/1 -> MATLAB Function3/2(q_dot)
  MATLAB Function3/1(w_b) -> w_GS/1
  v/1 -> MATLAB Function2/3(v)
  [C_IF] -> Matrix Multiply/1
